simulink model "three_phase_inverter"  (R2021a)
settings: Solver=ode45  StartTime=0.0  StopTime=0.5  RelTol=1e-3  EnableMultiTasking=on
values from neighbouring files (symbols this model uses):
  Cfilter = 40e-6    (= 4e-05)    [parameter.m]
  Lfilter = 2.4e-3    (= 0.0024)    [parameter.m]
  m = 0.95    [parameter.m]
  Res = 50    [parameter.m]
undefined symbols (not defined in the file or in its folder): i
libraries: spsIGBTDiodeLib x6, spsGroundLib x5, spsThreePhaseSeriesRLCBranchLib x3, spsCurrentMeasurementLib x3, spsThreePhaseVIMeasurementLib x2, spsDCVoltageSourceLib x2, spsPWMGenerator2LevelLib x1, simulink x1, spspowerguiLib x1
settings Model: Creator=TELE  LastModifiedBy=Kuhan
settings SolverCC: AlgebraicLoopSolver=TrustRegion
settings DataIOCC: LimitDataPoints=on  SaveFormat=Array  ReturnWorkspaceOutputs=off
settings OptimizationCC: LifeSpan=inf
settings DebuggingCC: UnderspecifiedInitializationDetection=Classic  MergeDetectMultiDrivingBlocksExec=none  SolverPrmCheckMsg=warning  StateNameClashWarn=warning  SFUnexpectedBacktrackingDiag=warning  SFNoUnconditionalDefaultTransitionDiag=warning  SFExecutionAtInitializationDiag=none  SFMachineParentedDataDiag=warning  ArithmeticOperatorsInVariantConditions=warning
settings HardwareCC: ProdBitPerPointer=32  ProdBitPerSizeT=32  ProdBitPerPtrDiffT=32  ProdLargestAtomicFloat=None  ProdIntDivRoundTo=Undefined  ProdEndianess=Unspecified  ProdWordSize=32  ProdHWDeviceType=32-bit Generic
settings ModelReferenceCC: PropagateSignalLabelsOutOfModel=off
settings SFSimCC: SimUseLocalCustomCode=off  CustomCodeUndefinedFunction=UseInterfaceOnly
settings RTWCC: RTWUseLocalCustomCode=off
settings CodeAppCC: StateflowObjectComments=on
settings GRTTargetCC: TargetLangStandard=C89/C90 (ANSI)
settings ConfigComp: CovMetricSettings=dw  CovSaveCumulativeToWorkspaceVar=on  CovSaveSingleToWorkspaceVar=on  CovExternalEMLEnable=off
settings SimscapeCC: SimscapeNormalizeSystem=off

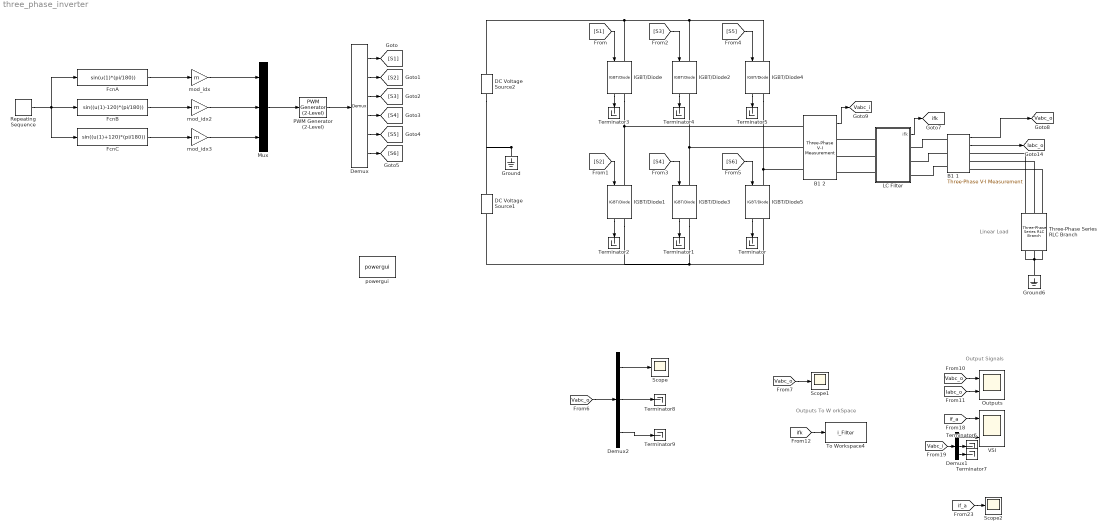
== system three_phase_inverter ==
  note: Linear Load
  note: Output Signals
  note: Outputs To W orkSpace
  B1 1 : spsThreePhaseVIMeasurementLib/Three-Phase V-I Measurement  VoltageMeasurement=phase-to-ground  SetLabelV=off  LabelV=Vabc  Vpu=off  VpuLL=off  CurrentMeasurement=yes  SetLabelI=off  LabelI=Iabc  Ipu=off  Pbase=100e6  Vbase=500e3  OutputType=Complex  PhasorSimulation=off  PSBequivalent=0
  B1 2 : spsThreePhaseVIMeasurementLib/Three-Phase V-I Measurement  VoltageMeasurement=phase-to-ground  SetLabelV=off  LabelV=Vabc  Vpu=off  VpuLL=off  CurrentMeasurement=no  SetLabelI=off  LabelI=Iabc  Ipu=off  Pbase=100e6  Vbase=500e3  OutputType=Complex  PhasorSimulation=off  PSBequivalent=0
  DC Voltage Source1 : spsDCVoltageSourceLib/DC Voltage Source  Amplitude=200  Measurements=None
  DC Voltage Source2 : spsDCVoltageSourceLib/DC Voltage Source  Amplitude=200  Measurements=None
  Demux : Demux  Outputs=6
  Demux1 : Demux  Outputs=3
  Demux2 : Demux  Outputs=3
  FcnA : Fcn  Expr=sin(u(1)*(pi/180))
  FcnB : Fcn  Expr=sin((u(1)-120)*(pi/180))
  FcnC : Fcn  Expr=sin((u(1)+120)*(pi/180))
  Ground : spsGroundLib/Ground  LConnTagsString=a
  Ground6 : spsGroundLib/Ground  LConnTagsString=a
  IGBT/Diode{,1..5} (6 alike) : spsIGBTDiodeLib/IGBT//Diode  Ron=1e-3  Rs=1e5  Cs=inf  Measurements=on
  LC Filter : Subsystem
  Mux : Mux  Inputs=3
  Outputs : Scope  NumInputPorts=2
  PWM Generator (2-Level) : spsPWMGenerator2LevelLib/PWM Generator (2-Level)  ModulatorType=Three-phase bridge (6 pulses)  ModulatorMode=Unsynchronized  Fc=27*50  Pc=90  nF=27  MinMax="[ -1  1 ]"  SamplingTechnique=Natural  ModulatingSignals=off  m=1  Freq=50  Phase=0  Ts=0  ShowCarrierOutport=off
  Repeating Sequence : simulink/Sources/Repeating Sequence  rep_seq_t=[0 1/50]  rep_seq_y=[0 360]
  Scope : Scope
  Scope1 : Scope
  Scope2 : Scope
  Terminator{,1..9} (10 alike) : Terminator
  Three-Phase Series RLC Branch : spsThreePhaseSeriesRLCBranchLib/Three-Phase Series RLC Branch  LConnTagsString=A|B|C  RConnTagsString=A|B|C  BranchType=R  Resistance=Res  Inductance=0.01  Capacitance=40e-6  Measurements=None
  To Workspace4 : ToWorkspace  VariableName=i_Filter  SampleTime=-1
  VSI : Scope  NumInputPorts=2
  "mod_idx " : Gain  Gain=m
  mod_idx2 : Gain  Gain=m
  mod_idx3 : Gain  Gain=m
  powergui : spspowerguiLib/powergui  Priority=1  SimulationMode=Discrete  SampleTime=50e-6  frequency=60  Iterations=50  frequencyindice=0  Pbase=100e6  ErrMax=1e-4  UnitsV=kV  UnitsW=MW  buscounter=0  FunctionMessages=off  echomessages=off  EnableUseOfTLC=off  CurrentSourceSwitches=off  DisableSnubberDevices=off  DisableRonSwitches=off  DisableVfSwitches=off  DisplayEquations=off  AutomaticDiscreteSolvers=off  SolverType=Tustin  Interpol=off  ExternalGateDelay=off  methode=off  Ts=0  x0status=blocks  SPID=off  SwTol=0  HookPort=off  NonlinearTolerance=1e-4  nMaxIteration=100  ContinueOnMaxIteration=off  RestoreLinks=warning  ResistiveCurrentMeasurement=off  Frange=[0:2:500]  Ylog=off  Xlog=on  ShowGrid=off  save=off  variable=ZData  structure=0  ZoomFFT=off  StartTime=0.0  cycles=1  DisplayStyle=1  fundamental=60  FreqAxis=off  MaxFrequency=1000  frequencyindicesteady=1  RmsSteady=1  display=off
  tag scope: Iabc_o=global, Vabc_i=global, Vabc_o=global, ifk=global
  wires:
  Demux/1 -> [S1]
  Demux/2 -> [S2]
  Demux/3 -> [S3]
  Demux/4 -> [S4]
  Demux/5 -> [S5]
  Demux/6 -> [S6]
  PWM Generator (2-Level)/1 -> Demux/1
  FcnA/1 -> "mod_idx "/1
  FcnB/1 -> mod_idx2/1
  FcnC/1 -> mod_idx3/1
  Mux/1 -> PWM Generator (2-Level)/1
  Repeating Sequence/1 -> FcnA/1, FcnC/1, FcnB/1
  "mod_idx "/1 -> Mux/1
  mod_idx2/1 -> Mux/2
  mod_idx3/1 -> Mux/3
  [S6] -> IGBT/Diode5/1
  IGBT/Diode5/1 -> Terminator/1
  IGBT/Diode/1 -> Terminator3/1
  [S1] -> IGBT/Diode/1
  IGBT/Diode2/1 -> Terminator4/1
  IGBT/Diode3/1 -> Terminator1/1
  [S4] -> IGBT/Diode3/1
  [S2] -> IGBT/Diode1/1
  [S5] -> IGBT/Diode4/1
  IGBT/Diode4/1 -> Terminator5/1
  [S3] -> IGBT/Diode2/1
  IGBT/Diode1/1 -> Terminator2/1
  B1 1/2 -> [Iabc_o]
  B1 2/1 -> [Vabc_i]
  LC Filter/1(ifk) -> [ifk]
  B1 1/1 -> [Vabc_o]
  Demux1/3 -> Terminator7/1
  [if_a] -> VSI/1
  Demux1/1 -> VSI/2
  Demux1/2 -> Terminator6/1
  [Vabc_o] -> Outputs/1
  [Vabc_i] -> Demux1/1
  [if_a] -> Scope2/1
  [Iabc_o] -> Outputs/2
  [ifk] -> To Workspace4/1
  [Vabc_o] -> Demux2/1
  Demux2/1 -> Scope/1
  Demux2/2 -> Terminator8/1
  Demux2/3 -> Terminator9/1
  [Vabc_o] -> Scope1/1
  connections:
  IGBT/Diode/RConn1 -- B1 2/LConn1 -- IGBT/Diode1/LConn1
  IGBT/Diode4/RConn1 -- B1 2/LConn3 -- IGBT/Diode5/LConn1
  IGBT/Diode/LConn1 -- DC Voltage Source2/RConn1 -- IGBT/Diode4/LConn1 -- IGBT/Diode2/LConn1
  Ground/LConn1 -- DC Voltage Source2/LConn1 -- DC Voltage Source1/RConn1
  IGBT/Diode3/RConn1 -- IGBT/Diode5/RConn1 -- IGBT/Diode1/RConn1 -- DC Voltage Source1/LConn1
  IGBT/Diode3/LConn1 -- IGBT/Diode2/RConn1 -- B1 2/LConn2
  Ground6/LConn1 -- Three-Phase Series RLC Branch/LConn1 -- Three-Phase Series RLC Branch/LConn2 -- Three-Phase Series RLC Branch/LConn3
  Three-Phase Series RLC Branch/RConn3 -- B1 1/RConn3
  B1 1/LConn3 -- LC Filter/RConn3
  LC Filter/LConn3 -- B1 2/RConn3
  B1 1/LConn2 -- LC Filter/RConn2
  LC Filter/LConn1 -- B1 2/RConn1
  Three-Phase Series RLC Branch/RConn1 -- B1 1/RConn1
  LC Filter/LConn2 -- B1 2/RConn2
  Three-Phase Series RLC Branch/RConn2 -- B1 1/RConn2
  B1 1/LConn1 -- LC Filter/RConn1

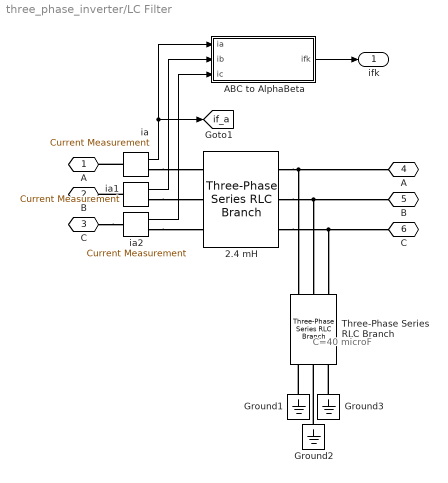
== system three_phase_inverter/LC Filter ==
  note: C=40 microF
  "2.4 mH " : spsThreePhaseSeriesRLCBranchLib/Three-Phase Series RLC Branch  LConnTagsString=A|B|C  RConnTagsString=A|B|C  BranchType=L  Resistance=1.0  Inductance=Lfilter  Capacitance=1.0  Measurements=None
  "ABC to AlphaBeta " : Subsystem
  Ground1 : spsGroundLib/Ground  LConnTagsString=a
  Ground2 : spsGroundLib/Ground  LConnTagsString=a
  Ground3 : spsGroundLib/Ground  LConnTagsString=a
  Three-Phase Series RLC Branch : spsThreePhaseSeriesRLCBranchLib/Three-Phase Series RLC Branch  LConnTagsString=A|B|C  RConnTagsString=A|B|C  BranchType=C  Resistance=1  Inductance=1e-3  Capacitance=Cfilter  Measurements=None
  ia : spsCurrentMeasurementLib/Current Measurement  PhasorSimulation=off  OutputType=Complex  PSBequivalent=0
  ia1 : spsCurrentMeasurementLib/Current Measurement  PhasorSimulation=off  OutputType=Complex  PSBequivalent=0
  ia2 : spsCurrentMeasurementLib/Current Measurement  PhasorSimulation=off  OutputType=Complex  PSBequivalent=0
  A : PMIOPort  Side=Left
  B : PMIOPort  Port=2  Side=Left
  C : PMIOPort  Port=3  Side=Left
  "A " : PMIOPort  Port=4  Side=Right
  "B " : PMIOPort  Port=5  Side=Right
  "C " : PMIOPort  Port=6  Side=Right
  ifk : Outport  VectorParamsAs1DForOutWhenUnconnected=off
  tag scope: if_a=global
  wires:
  ia/1 -> [if_a], "ABC to AlphaBeta "/1(ia)
  ia1/1 -> "ABC to AlphaBeta "/2(ib)
  ia2/1 -> "ABC to AlphaBeta "/3(ic)
  "ABC to AlphaBeta "/1(ifk) -> ifk/1
  connections:
  "2.4 mH "/RConn1 -- Three-Phase Series RLC Branch/RConn1 -- "A "/RConn1
  "2.4 mH "/RConn2 -- Three-Phase Series RLC Branch/RConn2 -- "B "/RConn1
  "2.4 mH "/RConn3 -- Three-Phase Series RLC Branch/RConn3 -- "C "/RConn1
  ia/LConn1 -- A/RConn1
  ia/RConn1 -- "2.4 mH "/LConn1
  ia1/LConn1 -- B/RConn1
  C/RConn1 -- ia2/LConn1
  ia1/RConn1 -- "2.4 mH "/LConn2
  ia2/RConn1 -- "2.4 mH "/LConn3
  Ground1/LConn1 -- Three-Phase Series RLC Branch/LConn1
  Ground2/LConn1 -- Three-Phase Series RLC Branch/LConn2
  Ground3/LConn1 -- Three-Phase Series RLC Branch/LConn3

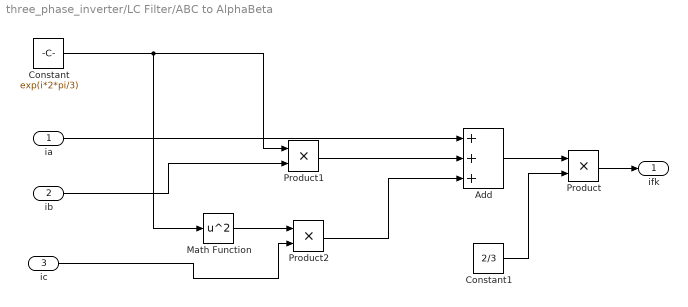
== system three_phase_inverter/LC Filter/ABC to AlphaBeta  ==
  ia : Inport
  ib : Inport  Port=2
  ic : Inport  Port=3
  Add : Sum  Inputs=+++
  Constant : Constant  Value=exp(i*2*pi/3)
  Constant1 : Constant  Value=2/3
  Math Function : Math  Operator=square  SignedPower=on  SaturateOnIntegerOverflow=on
  Product : Product  RndMeth=Zero
  Product1 : Product  RndMeth=Zero
  Product2 : Product  RndMeth=Zero
  ifk : Outport  VectorParamsAs1DForOutWhenUnconnected=off
  wires:
  Add/1 -> Product/1
  ia/1 -> Add/1
  Constant1/1 -> Product/2
  Product1/1 -> Add/2
  Constant/1 -> Product1/1, Math Function/1
  ib/1 -> Product1/2
  Math Function/1 -> Product2/1
  ic/1 -> Product2/2
  Product2/1 -> Add/3
  Product/1 -> ifk/1
